simulink model "SpatialContactForceBus"  (R2025a)
settings: Solver=ode45  StartTime=0.0  StopTime=10.0  MaxStep=1e-3  RelTol=1e-3  AbsTol=1e-3
PreLoadFcn:
  | addpath(fullfile('SpatialContactForceBusSupport','Scripts'));
model workspace: external: MATLAB File SpatialContactForceBusParameters.m (data not in the file)
undefined symbols (not defined in the file or in its folder): BackLeft, BackRight, BackStop, Body, car, critical_velocity, damping, EndRamp, FrontLeft, FrontRight, g, Incline, kinetic_friction_coef, LeftRail, Ramp1, Ramp2, Ramp3, Ramp4, ramp_structure, RightRail, static_friction_coef, stiffness, transition_region_width, X, Y, Z
libraries: sm_lib x131, SpatialContactForceBusLibrary x9, nesl_utility x1
(part 1 of 2)
CloseFcn:
  | rmpath(fullfile('SpatialContactForceBusSupport','Scripts'));
Description:
  | Using the Spatial Contact Force Block - Bumper Car
settings Model: Creator=The MathWorks, Inc.  LastModifiedBy=The MathWorks, Inc.
settings SolverCC: AutoScaleAbsTol=off  AlgebraicLoopSolver=TrustRegion
settings DataIOCC: ReturnWorkspaceOutputs=off
settings OptimizationCC: ReuseModelBlockBuffer=off
settings DebuggingCC: UnconnectedInputMsg=warning  UnconnectedOutputMsg=warning  UnconnectedLineMsg=warning  SubsystemReferenceDiagnosticForUnitTest=warning  SymbolicDimsDataTypeCodeGenerationDiagnostic=none
settings ModelReferenceCC: EnableRefExpFcnMdlSchedulingChecks=on
settings RTWCC: GPUComputeCapability=3.5
settings SimscapeCC: SimscapeLogType=all  SimscapeLogSimulationStatistics=on  SimscapeLogName=simlogSpatialContactForceBus  SimscapeLogDataHistory=20000.0
settings ExplorerConfigSet: InternalSimMechanicsExplorerSettings="<ExplorerConfiguration><canonicalview>default</canonicalview><AnimationSetting><BasePlaybackSpeed>1.0</BasePlaybackSpeed><PlaybackSpeedFactor>1.0</PlaybackSpeedFactor></AnimationSetting><TilePanel><TileInfo><Tiles Columns=\"1\" Count=\"1\" Rows=\"1\"><Column Weight=\"1\"/><Row Weight=\"1\"/><Tile Height=\"1\" Width=\"1\" X=\"0\" Y=\"0\"/></Tiles></TileInfo><SceneInfo><SceneViewer><BGColor><R>0.800000011920928955</R><G>0.800000011920928955</G><B>0.800000011920928955</B></BGColor><Camera><DoPerspective>off</DoPerspective><Position><X>0.637508295609907183</X><Y>-0.637508296451667844</Y><Z>1.11601012334107264</Z></Position><Center><X>-0.00639254054797280813</X><Y>0.00639253970621195267</Y><Z>0.472109287183192672</Z></Center><Up><X>-0.408248290463863073</X><Y>0.408248290463863073</Y><Z>0.816496580927726145</Z></Up><ViewLimDist>1</ViewLimDist><YLim>0.759088869094848628</YLim><XLim>0.995304530142192112</XLim></Camera></SceneViewer></SceneInfo></TilePanel><MechEditorPanel><Cameras/><GfxPanelCameraMap/><VideoCreator><PlaybackSpeedRatio>1.0</PlaybackSpeedRatio><FrameRate>30</FrameRate><VideoFormat>Motion JPEG AVI</VideoFormat><FrameSize>auto</FrameSize></VideoCreator></MechEditorPanel></ExplorerConfiguration>"

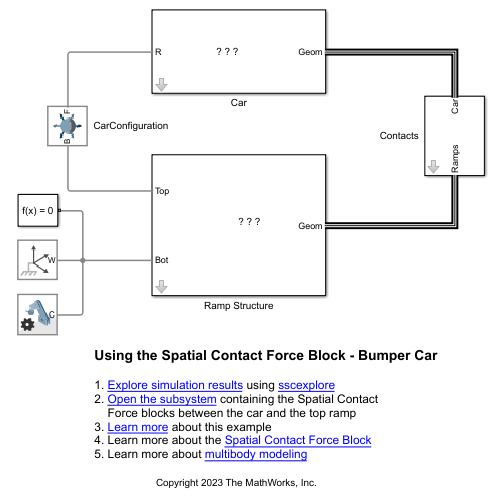
[thumbnail: Simulink's stored preview of the top-level diagram]
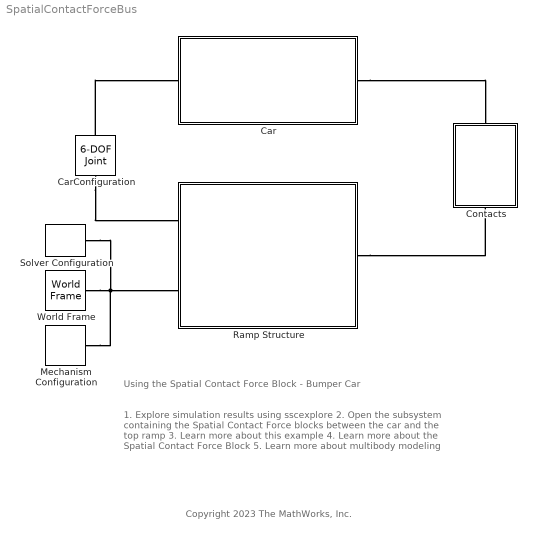
== system SpatialContactForceBus ==
  note: Copyright 2023 The MathWorks, Inc.
  note: Using the Spatial Contact Force Block - Bumper Car
  note: 1. Explore simulation results using sscexplore
      | 2. Open the subsystem containing the Spatial Contact
      | Force blocks between the car and the top ramp
      | 3. Learn more about this example
      | 4. Learn more about the Spatial Contact Force Block
      | 5. Learn more about multibody modeling
  Car : Subsystem  mask{l=car.body.length, w=car.body.width, h=car.body.height, m=car.body.mass, body_color=car.body.color, wheel_radius=car.wheel.radius, wheel_width=car.wheel.thickness, wheel_m=car.wheel.mass, wheel_color=car.wheel.color, wheel_spoke_color=car.wheel.spoke.color}
      mask prompts: l "Length (cm)"; w "Width (cm)"; h "Height (cm)"; m "Body Mass (kg)"; body_color "Car Body Color"; wheel_radius "Radius"; wheel_width "Thickness"; wheel_m "Wheel Mass (kg)"; wheel_color "Wheel Color"; wheel_spoke_color "Wheel Spoke Color"
      mask init:
      | axle_len               = .85 * l;
      | axle_radius            = axle_len / 30;
      | wheel_inner_radius     = .67 * wheel_radius;
      | wheel_spoke_thickness = axle_radius / 2;
      | 
      | front_wheel_pos  = l * .12;
      | back_wheel_pos   = l * .88;
      | wheel_separation = axle_len;
      mask DialogControl BodyGroupVar Prompt: Body
      mask DialogControl BodyDimGroupVar Prompt: Dimensions
      mask DialogControl BodyInertiaGroupVar Prompt: Inertia
      mask DialogControl BodyGraphicGroupVar Prompt: Graphic
      mask DialogControl WheelGroupVar Prompt: Wheels
      mask DialogControl WheelDimGroupVar Prompt: Dimensions
      mask DialogControl WheelInertiaGroupVar Prompt: Inertia
      mask DialogControl WheelGraphicGroupVar Prompt: Graphic
      mask Display: image(fullfile('SpatialContactForceBusSupport','Images','Car.png'));
  CarConfiguration : sm_lib/Joints/6-DOF Joint  JointMode=Normal  CompositeWrenchDir=FollowerOnBase  CompositeWrenchFrame=BaseFrame  SenseConstraintForce=off  SenseConstraintTorque=off  SenseTotalForce=off  SenseTotalTorque=off  PxPositionTargetSpecify=on  PxPositionTargetPriority=High  PxPositionTargetValue=car.start_dist  PxPositionTargetValueUnits=cm  PxVelocityTargetSpecify=off  PxVelocityTargetPriority=High  PxVelocityTargetValue=0  PxVelocityTargetValueUnits=m/s  PxEquilibriumPosition=0  PxEquilibriumPositionUnits=m  PxSpringStiffness=0  PxSpringStiffnessUnits=N/m  PxDampingCoefficient=0  PxDampingCoefficientUnits=N/(m/s)  PxLowerLimitSpecify=off  PxLowerLimitBound=-1  PxLowerLimitBoundUnits=m  PxLowerLimitStiffness=1e6  PxLowerLimitStiffnessUnits=N/m  PxLowerLimitDamping=1e3  PxLowerLimitDampingUnits=N/(m/s)  PxLowerLimitTransitionRegionWidth=1e-4  PxLowerLimitTransitionRegionWidthUnits=m  PxUpperLimitSpecify=off  PxUpperLimitBound=1  PxUpperLimitBoundUnits=m  PxUpperLimitStiffness=1e6  PxUpperLimitStiffnessUnits=N/m  PxUpperLimitDamping=1e3  PxUpperLimitDampingUnits=N/(m/s)  PxUpperLimitTransitionRegionWidth=1e-4  PxUpperLimitTransitionRegionWidthUnits=m  PxTorqueActuationMode=NoTorque  PxMotionActuationMode=ComputedMotion  PxSensePosition=off  PxSenseVelocity=off  PxSenseAcceleration=off  PxSenseTorqueForce=off  PxSenseLowerLimitTorqueForce=off  PxSenseUpperLimitTorqueForce=off  PyPositionTargetSpecify=off  PyPositionTargetPriority=High  PyPositionTargetValue=0  PyPositionTargetValueUnits=m  PyVelocityTargetSpecify=off  PyVelocityTargetPriority=High  PyVelocityTargetValue=0  PyVelocityTargetValueUnits=m/s  PyEquilibriumPosition=0  PyEquilibriumPositionUnits=m  PySpringStiffness=0  PySpringStiffnessUnits=N/m  PyDampingCoefficient=0  PyDampingCoefficientUnits=N/(m/s)  PyLowerLimitSpecify=off  PyLowerLimitBound=-1  PyLowerLimitBoundUnits=m  PyLowerLimitStiffness=1e6  PyLowerLimitStiffnessUnits=N/m  PyLowerLimitDamping=1e3  PyLowerLimitDampingUnits=N/(m/s)  PyLowerLimitTransitionRegionWidth=1e-4  PyLowerLimitTransitionRegionWidthUnits=m  PyUpperLimitSpecify=off  PyUpperLimitBound=1  PyUpperLimitBoundUnits=m  PyUpperLimitStiffness=1e6  PyUpperLimitStiffnessUnits=N/m  PyUpperLimitDamping=1e3  PyUpperLimitDampingUnits=N/(m/s)  PyUpperLimitTransitionRegionWidth=1e-4  PyUpperLimitTransitionRegionWidthUnits=m  PyTorqueActuationMode=NoTorque  PyMotionActuationMode=ComputedMotion  PySensePosition=off  PySenseVelocity=off  PySenseAcceleration=off  PySenseTorqueForce=off  PySenseLowerLimitTorqueForce=off  PySenseUpperLimitTorqueForce=off  PzPositionTargetSpecify=on  PzPositionTargetPriority=High  PzPositionTargetValue=car.start_height  PzPositionTargetValueUnits=cm  PzVelocityTargetSpecify=off  PzVelocityTargetPriority=High  PzVelocityTargetValue=0  PzVelocityTargetValueUnits=m/s  PzEquilibriumPosition=0  PzEquilibriumPositionUnits=m  PzSpringStiffness=0  PzSpringStiffnessUnits=N/m  PzDampingCoefficient=0  PzDampingCoefficientUnits=N/(m/s)  PzLowerLimitSpecify=off  PzLowerLimitBound=-1  PzLowerLimitBoundUnits=m  PzLowerLimitStiffness=1e6  PzLowerLimitStiffnessUnits=N/m  PzLowerLimitDamping=1e3  PzLowerLimitDampingUnits=N/(m/s)  PzLowerLimitTransitionRegionWidth=1e-4  PzLowerLimitTransitionRegionWidthUnits=m  PzUpperLimitSpecify=off  PzUpperLimitBound=1  PzUpperLimitBoundUnits=m  PzUpperLimitStiffness=1e6  PzUpperLimitStiffnessUnits=N/m  PzUpperLimitDamping=1e3  PzUpperLimitDampingUnits=N/(m/s)  PzUpperLimitTransitionRegionWidth=1e-4  PzUpperLimitTransitionRegionWidthUnits=m  PzTorqueActuationMode=NoTorque  PzMotionActuationMode=ComputedMotion  PzSensePosition=off  PzSenseVelocity=off  PzSenseAcceleration=off  PzSenseTorqueForce=off  PzSenseLowerLimitTorqueForce=off  PzSenseUpperLimitTorqueForce=off  SphPositionTargetSpecify=on  SphPositionTargetPriority=High  SphPositionTargetRotationMethod=StandardAxis  SphPositionTargetFollAlignAxisA=+X  SphPositionTargetBaseAlignAxisA=+Y  SphPositionTargetFollAlignAxisB=+Y  SphPositionTargetBaseAlignAxisB=+Z  SphPositionTargetRotationStandardAxis=-Y  SphPositionTargetRotationAngle=car.start_pitch  SphPositionTargetRotationAngleUnits=deg  SphPositionTargetRotationArbitraryAxis=[0 0 1]  SphPositionTargetRotationSequenceAxes=FollowerAxes  SphPositionTargetRotationSequence=XYX  SphPositionTargetRotationSequenceAngles=[0 0 0]  SphPositionTargetRotationSequenceAnglesUnits=deg  SphPositionTargetRotationMatrix=[1 0 0; 0 1 0; 0 0 1]  SphPositionTargetQuaternion=[1 0 0 0]  SphVelocityTargetSpecify=off  SphVelocityTargetPriority=High  SphVelocityTargetValue=[0 0 0]  SphVelocityTargetValueUnits=deg/s  SphVelocityTargetInFollowerFrame=on  SphEqPosRotationMethod=None  SphEqPosFollAlignAxisA=+X  SphEqPosBaseAlignAxisA=+Y  SphEqPosFollAlignAxisB=+Y  SphEqPosBaseAlignAxisB=+Z  SphEqPosRotationStandardAxis=+Z  SphEqPosRotationAngle=0.0  SphEqPosRotationAngleUnits=deg  SphEqPosRotationArbitraryAxis=[0 0 1]  SphEqPosRotationSequenceAxes=FollowerAxes  SphEqPosRotationSequence=XYX  SphEqPosRotationSequenceAngles=[0 0 0]  SphEqPosRotationSequenceAnglesUnits=deg  SphEqPosRotationMatrix=[1 0 0; 0 1 0; 0 0 1]  SphEqPosQuaternion=[1 0 0 0]  SphSpringStiffness=0  SphSpringStiffnessUnits=N*m/deg  SphDampingCoefficient=0  SphDampingCoefficientUnits=N*m/(deg/s)  SphLowerLimitSpecify=off  SphLowerLimitBound=15  SphLowerLimitBoundUnits=deg  SphLowerLimitStiffness=1e4  SphLowerLimitStiffnessUnits=N*m/deg  SphLowerLimitDamping=10  SphLowerLimitDampingUnits=N*m/(deg/s)  SphLowerLimitTransitionRegionWidth=0.1  SphLowerLimitTransitionRegionWidthUnits=deg  SphUpperLimitSpecify=off  SphUpperLimitBound=45  SphUpperLimitBoundUnits=deg  SphUpperLimitStiffness=1e4  SphUpperLimitStiffnessUnits=N*m/deg  SphUpperLimitDamping=10  SphUpperLimitDampingUnits=N*m/(deg/s)  SphUpperLimitTransitionRegionWidth=0.1  SphUpperLimitTransitionRegionWidthUnits=deg  SphTorqueActuationMode=NoTorque  SphActuateTorqueX=off  SphActuateTorqueY=off  SphActuateTorqueZ=off  SphActuateTorque=off  SphActuationFrame=BaseFrame  SphSensePosition=off  SphSenseVelocityX=off  SphSenseVelocityY=off  SphSenseVelocityZ=off  SphSenseVelocity=off  SphSenseAccelerationX=off  SphSenseAccelerationY=off  SphSenseAccelerationZ=off  SphSenseAcceleration=off  SphSenseLowerLimitTorqueMag=off  SphSenseUpperLimitTorqueMag=off  SphSensingFrame=BaseFrame
  Contacts : Subsystem  mask{k=stiffness, b=damping, tau=transition_region_width, mus=static_friction_coef, muk=kinetic_friction_coef, cv=critical_velocity}
      mask prompts: k "Stiffness (N/m)"; b "Damping (N/(m/s))"; tau "Transition Region Width (m)"; mus "Coefficient of Static Friction"; muk "Coefficient of Kinetic Friction"; cv "Critical Velocity (m/s)"
  Mechanism Configuration : sm_lib/Utilities/Mechanism Configuration  UniformGravity=Constant  GravityVector=[0 0 -g]  GravityVectorUnits=m/s^2  LinearizationDelta=0.001  JointModeTransitionNonlinearIterations=2
  Ramp Structure : Subsystem  mask{w=ramp_structure.width, l=ramp_structure.length, ramp_angle=ramp_structure.ramp.angle, surface_color=ramp_structure.ramp.color, rail_color=ramp_structure.rail.color, pillar_color=ramp_structure.pillar.color, base_color=ramp_structure.base.color}
      mask prompts: w "Width (cm)"; l "Length (cm)"; ramp_angle "Ramp Angle (deg)"; surface_color "Surface Color"; rail_color "Rail Color"; pillar_color "Pillar Color"; base_color "Base Color"
      mask init:
      | ramp.angle = ramp_angle;
      | theta_ = deg2rad(ramp.angle);
      | 
      | ramp.w       = w;
      | ramp.h       = ramp.w / 4;
      | 
      | wall.h        = ramp.w;
      | 
      | dropoff_h     = .75 * ramp.w;
      | dropoff_dist  = 1.5 * ramp.w;
      | 
      | ramp.l        = (l - dropoff_dist - sin(theta_)*ramp.h/2)...
      |                 / cos(theta_);
      | 
      | rail.r        = .28 * ramp.h;
      | rail.l        = ramp.l;
      | 
      | rail.h = 1.5 * ramp.h;
      | 
      | end_ramp.l = dropoff_dist + ramp.h;
      | 
      | ramp.w = ramp.w + 2 * rail.r;
      mask DialogControl ParameterGroupVar Prompt: Geometry
      mask DialogControl GraphicsGroupVar Prompt: Graphic
      mask Display: image(fullfile('SpatialContactForceBusSupport','Images','RampStructure.png'));
  Solver Configuration : nesl_utility/Solver Configuration  PhysicalDomain=network_engine_domain  SubClassName=solver  LeftPortType=input  RightPortType=generic  Tones=[]  Harmonics=[]  SimulateNoise=off  Profile=off  UseLocalSampling=off  EnableSwitchedLinearOptims=on  FrequencyDomain=off  UseCCode=off  RelTol=0.001  AbsTol=1e-06  MinStep=1e-09  ToWorkspace=off  RevertToSquareIcSolve=off  NumHomotopyIterations=100  PhasorMode=off  PhasorModeNumHarmonics=1  ConsistencySolver=NEWTON_FTOL  IndexReductionMethod=DerivativeReplacement  DoDC=off  ResidualTolerance=1e-09  ConsistencyTolSource=GLOBAL  ConsistencyAbsTol=0.001  ConsistencyRelTol=0.001  ConsistencyTolFactor=0.001  UseLocalSolver=off  LocalSolverChoice=NE_BACKWARD_EULER_ADVANCER  ResolveIndetEquations=on  FunctionEvalNumThread=1  LocalSolverSampleTime=0.001  DoFixedCost=off  MaxNonlinIter=3  MaxModeIter=2  ComputeImpulses=off  ImpulseIterations=2  LinearAlgebra=Sparse  LinearAlgebraNumThread=0  EquationFormulation=NE_TIME_EF  DelaysMemoryBudget=1024  AutomaticFiltering=on  FilteringTimeConstant=0.001  PartitionStorageMethod=AS_NEEDED  PartitionMemoryBudget=1024  PartitionMethod=FAST  MultibodyUseLocalSolver=off  MultibodyLocalSolverChoice=ODE1  MultibodyLocalSolverSampleTime=0.001
  World Frame : sm_lib/Frames and Transforms/World Frame
  connections:
  Solver Configuration/RConn1 -- Ramp Structure/LConn2 -- Mechanism Configuration/RConn1 -- World Frame/RConn1
  CarConfiguration/RConn1 -- Car/LConn1
  CarConfiguration/LConn1 -- Ramp Structure/LConn1
  Ramp Structure/RConn1 -- Contacts/LConn1
  Car/RConn1 -- Contacts/RConn1

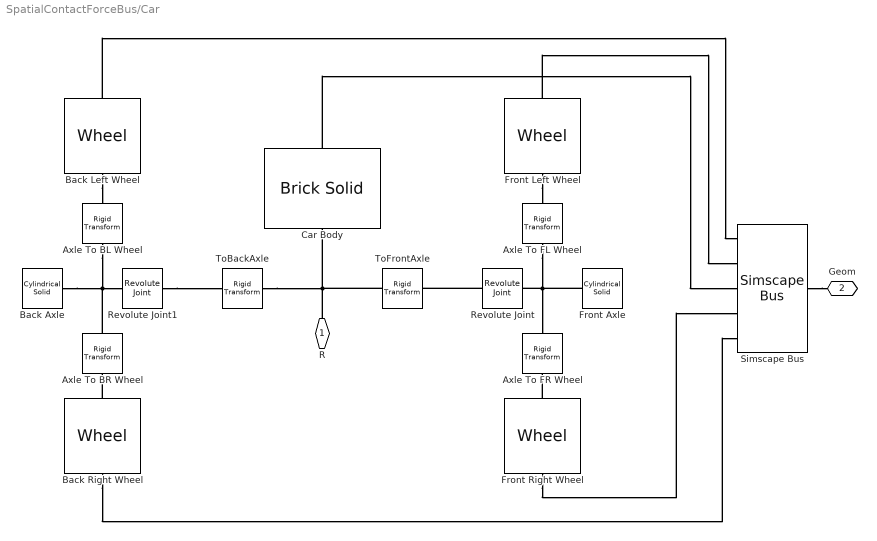
== system SpatialContactForceBus/Car ==
  Axle To BL Wheel : sm_lib/Frames and Transforms/Rigid Transform  RotationMethod=None  FollAlignAxisA=+X  BaseAlignAxisA=+Y  FollAlignAxisB=+Y  BaseAlignAxisB=+Z  RotationStandardAxis=+Z  RotationAngle=0.0  RotationAngleUnits=deg  RotationArbitraryAxis=[0 0 1]  RotationSequenceAxes=FollowerAxes  RotationSequence=XYX  RotationSequenceAngles=[0 0 0]  RotationSequenceAnglesUnits=deg  RotationMatrix=[1 0 0; 0 1 0; 0 0 1]  Quaternion=[1 0 0 0]  TranslationMethod=StandardAxis  TranslationCartesianOffset=[0 0 0]  TranslationCartesianOffsetUnits=cm  TranslationStandardAxis=-Z  TranslationStandardOffset=wheel_separation/2  TranslationStandardOffsetUnits=cm  TranslationROffset=0  TranslationROffsetUnits=m  TranslationThetaOffset=0  TranslationThetaOffsetUnits=deg  TranslationZOffset=0  TranslationZOffsetUnits=m
  Axle To BR Wheel : sm_lib/Frames and Transforms/Rigid Transform  RotationMethod=None  FollAlignAxisA=+X  BaseAlignAxisA=+Y  FollAlignAxisB=+Y  BaseAlignAxisB=+Z  RotationStandardAxis=+Z  RotationAngle=0.0  RotationAngleUnits=deg  RotationArbitraryAxis=[0 0 1]  RotationSequenceAxes=FollowerAxes  RotationSequence=XYX  RotationSequenceAngles=[0 0 0]  RotationSequenceAnglesUnits=deg  RotationMatrix=[1 0 0; 0 1 0; 0 0 1]  Quaternion=[1 0 0 0]  TranslationMethod=StandardAxis  TranslationCartesianOffset=[0 0 0]  TranslationCartesianOffsetUnits=cm  TranslationStandardAxis=+Z  TranslationStandardOffset=wheel_separation/2  TranslationStandardOffsetUnits=cm  TranslationROffset=0  TranslationROffsetUnits=m  TranslationThetaOffset=0  TranslationThetaOffsetUnits=deg  TranslationZOffset=0  TranslationZOffsetUnits=m
  Axle To FL Wheel : sm_lib/Frames and Transforms/Rigid Transform  RotationMethod=None  FollAlignAxisA=+X  BaseAlignAxisA=+Y  FollAlignAxisB=+Y  BaseAlignAxisB=+Z  RotationStandardAxis=+Z  RotationAngle=0.0  RotationAngleUnits=deg  RotationArbitraryAxis=[0 0 1]  RotationSequenceAxes=FollowerAxes  RotationSequence=XYX  RotationSequenceAngles=[0 0 0]  RotationSequenceAnglesUnits=deg  RotationMatrix=[1 0 0; 0 1 0; 0 0 1]  Quaternion=[1 0 0 0]  TranslationMethod=StandardAxis  TranslationCartesianOffset=[0 0 0]  TranslationCartesianOffsetUnits=cm  TranslationStandardAxis=-Z  TranslationStandardOffset=wheel_separation/2  TranslationStandardOffsetUnits=cm  TranslationROffset=0  TranslationROffsetUnits=m  TranslationThetaOffset=0  TranslationThetaOffsetUnits=deg  TranslationZOffset=0  TranslationZOffsetUnits=m
  Axle To FR Wheel : sm_lib/Frames and Transforms/Rigid Transform  RotationMethod=None  FollAlignAxisA=+X  BaseAlignAxisA=+Y  FollAlignAxisB=+Y  BaseAlignAxisB=+Z  RotationStandardAxis=+Z  RotationAngle=0.0  RotationAngleUnits=deg  RotationArbitraryAxis=[0 0 1]  RotationSequenceAxes=FollowerAxes  RotationSequence=XYX  RotationSequenceAngles=[0 0 0]  RotationSequenceAnglesUnits=deg  RotationMatrix=[1 0 0; 0 1 0; 0 0 1]  Quaternion=[1 0 0 0]  TranslationMethod=StandardAxis  TranslationCartesianOffset=[0 0 0]  TranslationCartesianOffsetUnits=cm  TranslationStandardAxis=+Z  TranslationStandardOffset=wheel_separation/2  TranslationStandardOffsetUnits=cm  TranslationROffset=0  TranslationROffsetUnits=m  TranslationThetaOffset=0  TranslationThetaOffsetUnits=deg  TranslationZOffset=0  TranslationZOffsetUnits=m
  Back Axle : sm_lib/Body Elements/Cylindrical Solid  CylinderRadius=axle_radius  CylinderRadiusUnits=cm  CylinderLength=axle_len  CylinderLengthUnits=cm  ExportEntireGeometry=off  InertiaType=CalculateFromGeometry  BasedOnType=Density  Density=0  DensityUnits=kg/m^3  Mass=1  MassUnits=kg  CenterOfMass=[0 0 0]  CenterOfMassUnits=m  MomentsOfInertia=[1 1 1]  MomentsOfInertiaUnits=kg*m^2  ProductsOfInertia=[0 0 0]  ProductsOfInertiaUnits=kg*m^2  GraphicType=FromGeometry  MarkerShape=Sphere  MarkerSize=10  GraphicVisPropType=SimpleVisualProperties  GraphicDiffuseColor=wheel_spoke_color  GraphicOpacity=1.0  GraphicSpecularColor=[0.5 0.5 0.5 1.0]  GraphicAmbientColor=[0.15 0.15 0.15 1.0]  GraphicEmissiveColor=[0.0 0.0 0.0 1.0]  GraphicShininess=75  DoExposeReferenceFrame=on  SerializedFrames=<Frames/>
  Back Left Wheel : SpatialContactForceBusLibrary/Wheel  r=wheel_radius  rin=wheel_inner_radius  spoke_r=wheel_spoke_thickness  W=wheel_width  m=wheel_m  color=wheel_color  spoke_color=wheel_spoke_color
  Back Right Wheel : SpatialContactForceBusLibrary/Wheel  r=wheel_radius  rin=wheel_inner_radius  spoke_r=wheel_spoke_thickness  W=wheel_width  m=wheel_m  color=wheel_color  spoke_color=wheel_spoke_color
  Car Body : sm_lib/Body Elements/Brick Solid  BrickDimensions=[l w h]  BrickDimensionsUnits=cm  ExportEntireGeometry=on  InertiaType=CalculateFromGeometry  BasedOnType=Mass  Density=1000  DensityUnits=kg/m^3  Mass=m  MassUnits=kg  CenterOfMass=[0 0 0]  CenterOfMassUnits=cm  MomentsOfInertia=[1 1 1]  MomentsOfInertiaUnits=kg*m^2  ProductsOfInertia=[0 0 0]  ProductsOfInertiaUnits=kg*m^2  GraphicType=FromGeometry  MarkerShape=Sphere  MarkerSize=10  GraphicVisPropType=SimpleVisualProperties  GraphicDiffuseColor=body_color  GraphicOpacity=1.0  GraphicSpecularColor=[0.5 0.5 0.5 1.0]  GraphicAmbientColor=[0.15 0.15 0.15 1.0]  GraphicEmissiveColor=[0.0 0.0 0.0 1.0]  GraphicShininess=75  DoExposeReferenceFrame=on  SerializedFrames=<Frames/>
  Front Axle : sm_lib/Body Elements/Cylindrical Solid  CylinderRadius=axle_radius  CylinderRadiusUnits=cm  CylinderLength=axle_len  CylinderLengthUnits=cm  ExportEntireGeometry=off  InertiaType=CalculateFromGeometry  BasedOnType=Density  Density=0  DensityUnits=kg/m^3  Mass=1  MassUnits=kg  CenterOfMass=[0 0 0]  CenterOfMassUnits=m  MomentsOfInertia=[1 1 1]  MomentsOfInertiaUnits=kg*m^2  ProductsOfInertia=[0 0 0]  ProductsOfInertiaUnits=kg*m^2  GraphicType=FromGeometry  MarkerShape=Sphere  MarkerSize=10  GraphicVisPropType=SimpleVisualProperties  GraphicDiffuseColor=wheel_spoke_color  GraphicOpacity=1.0  GraphicSpecularColor=[0.5 0.5 0.5 1.0]  GraphicAmbientColor=[0.15 0.15 0.15 1.0]  GraphicEmissiveColor=[0.0 0.0 0.0 1.0]  GraphicShininess=75  DoExposeReferenceFrame=on  SerializedFrames=<Frames/>
  Front Left Wheel : SpatialContactForceBusLibrary/Wheel  r=wheel_radius  rin=wheel_inner_radius  spoke_r=wheel_spoke_thickness  W=wheel_width  m=wheel_m  color=wheel_color  spoke_color=wheel_spoke_color
  Front Right Wheel : SpatialContactForceBusLibrary/Wheel  r=wheel_radius  rin=wheel_inner_radius  spoke_r=wheel_spoke_thickness  W=wheel_width  m=wheel_m  color=wheel_color  spoke_color=wheel_spoke_color
  Revolute Joint : sm_lib/Joints/Revolute Joint  JointMode=Normal  CompositeWrenchDir=FollowerOnBase  CompositeWrenchFrame=BaseFrame  SenseConstraintForce=off  SenseConstraintTorque=off  SenseTotalForce=off  SenseTotalTorque=off  PositionTargetSpecify=off  PositionTargetPriority=High  PositionTargetValue=0  PositionTargetValueUnits=deg  VelocityTargetSpecify=off  VelocityTargetPriority=High  VelocityTargetValue=0  VelocityTargetValueUnits=deg/s  EquilibriumPosition=0  EquilibriumPositionUnits=deg  SpringStiffness=0  SpringStiffnessUnits=N*m/deg  DampingCoefficient=0  DampingCoefficientUnits=N*m/(deg/s)  LowerLimitSpecify=off  LowerLimitBound=-90  LowerLimitBoundUnits=deg  LowerLimitStiffness=1e4  LowerLimitStiffnessUnits=N*m/deg  LowerLimitDamping=10  LowerLimitDampingUnits=N*m/(deg/s)  LowerLimitTransitionRegionWidth=0.1  LowerLimitTransitionRegionWidthUnits=deg  UpperLimitSpecify=off  UpperLimitBound=90  UpperLimitBoundUnits=deg  UpperLimitStiffness=1e4  UpperLimitStiffnessUnits=N*m/deg  UpperLimitDamping=10  UpperLimitDampingUnits=N*m/(deg/s)  UpperLimitTransitionRegionWidth=0.1  UpperLimitTransitionRegionWidthUnits=deg  TorqueActuationMode=NoTorque  MotionActuationMode=ComputedMotion  SensePosition=off  SenseVelocity=off  SenseAcceleration=off  SenseTorqueForce=off  SenseLowerLimitTorqueForce=off  SenseUpperLimitTorqueForce=off
  Revolute Joint1 : sm_lib/Joints/Revolute Joint  JointMode=Normal  CompositeWrenchDir=FollowerOnBase  CompositeWrenchFrame=BaseFrame  SenseConstraintForce=off  SenseConstraintTorque=off  SenseTotalForce=off  SenseTotalTorque=off  PositionTargetSpecify=off  PositionTargetPriority=High  PositionTargetValue=0  PositionTargetValueUnits=deg  VelocityTargetSpecify=off  VelocityTargetPriority=High  VelocityTargetValue=0  VelocityTargetValueUnits=deg/s  EquilibriumPosition=0  EquilibriumPositionUnits=deg  SpringStiffness=0  SpringStiffnessUnits=N*m/deg  DampingCoefficient=0  DampingCoefficientUnits=N*m/(deg/s)  LowerLimitSpecify=off  LowerLimitBound=-90  LowerLimitBoundUnits=deg  LowerLimitStiffness=1e4  LowerLimitStiffnessUnits=N*m/deg  LowerLimitDamping=10  LowerLimitDampingUnits=N*m/(deg/s)  LowerLimitTransitionRegionWidth=0.1  LowerLimitTransitionRegionWidthUnits=deg  UpperLimitSpecify=off  UpperLimitBound=90  UpperLimitBoundUnits=deg  UpperLimitStiffness=1e4  UpperLimitStiffnessUnits=N*m/deg  UpperLimitDamping=10  UpperLimitDampingUnits=N*m/(deg/s)  UpperLimitTransitionRegionWidth=0.1  UpperLimitTransitionRegionWidthUnits=deg  TorqueActuationMode=NoTorque  MotionActuationMode=ComputedMotion  SensePosition=off  SenseVelocity=off  SenseAcceleration=off  SenseTorqueForce=off  SenseLowerLimitTorqueForce=off  SenseUpperLimitTorqueForce=off
  Simscape Bus : SimscapeBus  HierarchyStrings=BackLeft;FrontLeft;Body;FrontRight;BackRight
  ToBackAxle : sm_lib/Frames and Transforms/Rigid Transform  RotationMethod=AlignedAxes  FollAlignAxisA=+Y  BaseAlignAxisA=+Z  FollAlignAxisB=+Z  BaseAlignAxisB=-Y  RotationStandardAxis=+Z  RotationAngle=0.0  RotationAngleUnits=deg  RotationArbitraryAxis=[0 0 1]  RotationSequenceAxes=FollowerAxes  RotationSequence=XYX  RotationSequenceAngles=[0 0 0]  RotationSequenceAnglesUnits=deg  RotationMatrix=[1 0 0; 0 1 0; 0 0 1]  Quaternion=[1 0 0 0]  TranslationMethod=StandardAxis  TranslationCartesianOffset=[0 0 0]  TranslationCartesianOffsetUnits=cm  TranslationStandardAxis=+X  TranslationStandardOffset=l/2 - back_wheel_pos  TranslationStandardOffsetUnits=cm  TranslationROffset=0  TranslationROffsetUnits=m  TranslationThetaOffset=0  TranslationThetaOffsetUnits=deg  TranslationZOffset=0  TranslationZOffsetUnits=m
  ToFrontAxle : sm_lib/Frames and Transforms/Rigid Transform  RotationMethod=AlignedAxes  FollAlignAxisA=+Y  BaseAlignAxisA=+Z  FollAlignAxisB=+Z  BaseAlignAxisB=-Y  RotationStandardAxis=+Z  RotationAngle=0.0  RotationAngleUnits=deg  RotationArbitraryAxis=[0 0 1]  RotationSequenceAxes=FollowerAxes  RotationSequence=XYX  RotationSequenceAngles=[0 0 0]  RotationSequenceAnglesUnits=deg  RotationMatrix=[1 0 0; 0 1 0; 0 0 1]  Quaternion=[1 0 0 0]  TranslationMethod=StandardAxis  TranslationCartesianOffset=[0 0 0]  TranslationCartesianOffsetUnits=cm  TranslationStandardAxis=+X  TranslationStandardOffset=l/2 - front_wheel_pos  TranslationStandardOffsetUnits=cm  TranslationROffset=0  TranslationROffsetUnits=m  TranslationThetaOffset=0  TranslationThetaOffsetUnits=deg  TranslationZOffset=0  TranslationZOffsetUnits=m
  R : PMIOPort  Side=Left
  Geom : PMIOPort  Port=2  Side=Right
  connections:
  Back Right Wheel/LConn1 -- Axle To BR Wheel/RConn1
  ToFrontAxle/LConn1 -- Car Body/RConn1 -- R/RConn1 -- ToBackAxle/LConn1
  Front Left Wheel/LConn1 -- Axle To FL Wheel/RConn1
  Revolute Joint1/LConn1 -- ToBackAxle/RConn1
  Revolute Joint/LConn1 -- ToFrontAxle/RConn1
  Axle To FL Wheel/LConn1 -- Front Axle/RConn1 -- Axle To FR Wheel/LConn1 -- Revolute Joint/RConn1
  Axle To BR Wheel/LConn1 -- Back Axle/RConn1 -- Axle To BL Wheel/LConn1 -- Revolute Joint1/RConn1
  Front Right Wheel/LConn1 -- Axle To FR Wheel/RConn1
  Back Left Wheel/LConn1 -- Axle To BL Wheel/RConn1
  Simscape Bus/RConn1 -- Geom/RConn1
  Car Body/LConn1 -- Simscape Bus/LConn3
  Front Left Wheel/RConn1 -- Simscape Bus/LConn2
  Back Left Wheel/RConn1 -- Simscape Bus/LConn1
  Front Right Wheel/RConn1 -- Simscape Bus/LConn4
  Back Right Wheel/RConn1 -- Simscape Bus/LConn5

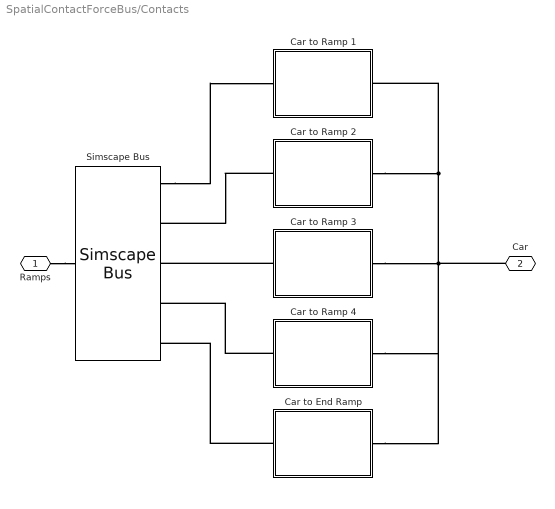
== system SpatialContactForceBus/Contacts ==
  Car to End Ramp : Subsystem
  Car to Ramp 1 : Subsystem
  Car to Ramp 2 : Subsystem
  Car to Ramp 3 : Subsystem
  Car to Ramp 4 : Subsystem
  Simscape Bus : SimscapeBus  HierarchyStrings=Ramp1;Ramp2;Ramp3;Ramp4;EndRamp
  Ramps : PMIOPort  Side=Left
  Car : PMIOPort  Port=2  Side=Right
  connections:
  Ramps/RConn1 -- Simscape Bus/RConn1
  Simscape Bus/LConn1 -- Car to Ramp 1/LConn1
  Car to Ramp 2/LConn1 -- Simscape Bus/LConn2
  Car to Ramp 3/LConn1 -- Simscape Bus/LConn3
  Car to Ramp 4/LConn1 -- Simscape Bus/LConn4
  Car to End Ramp/LConn1 -- Simscape Bus/LConn5
  Car/RConn1 -- Car to Ramp 3/RConn1 -- Car to End Ramp/RConn1 -- Car to Ramp 4/RConn1 -- Car to Ramp 2/RConn1 -- Car to Ramp 1/RConn1

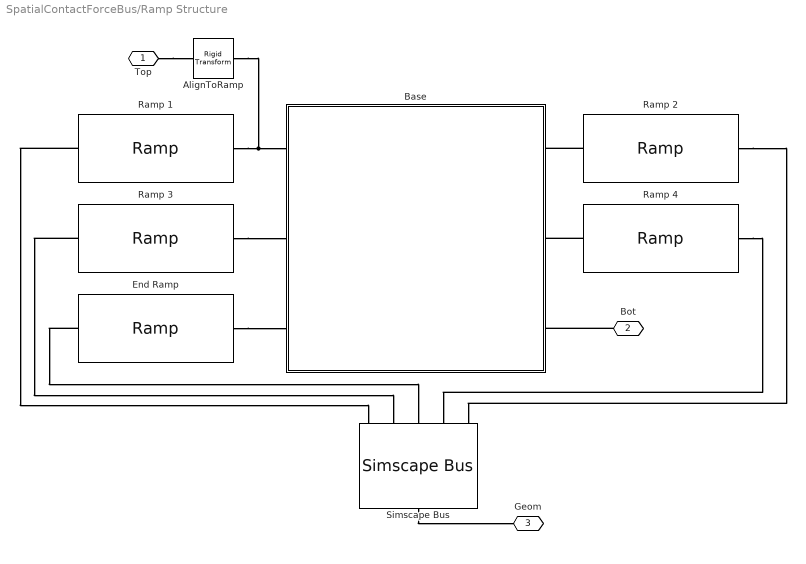
== system SpatialContactForceBus/Ramp Structure ==
  AlignToRamp : sm_lib/Frames and Transforms/Rigid Transform  RotationMethod=StandardAxis  FollAlignAxisA=+X  BaseAlignAxisA=+Y  FollAlignAxisB=+Y  BaseAlignAxisB=+Z  RotationStandardAxis=+Y  RotationAngle=ramp_angle  RotationAngleUnits=deg  RotationArbitraryAxis=[0 0 1]  RotationSequenceAxes=FollowerAxes  RotationSequence=XYX  RotationSequenceAngles=[0 0 0]  RotationSequenceAnglesUnits=deg  RotationMatrix=[1 0 0; 0 1 0; 0 0 1]  Quaternion=[1 0 0 0]  TranslationMethod=None  TranslationCartesianOffset=[0 0 0]  TranslationCartesianOffsetUnits=cm  TranslationStandardAxis=+Z  TranslationStandardOffset=0  TranslationStandardOffsetUnits=cm  TranslationROffset=0  TranslationROffsetUnits=m  TranslationThetaOffset=0  TranslationThetaOffsetUnits=deg  TranslationZOffset=0  TranslationZOffsetUnits=m
  Base : Subsystem  mask{width=w, length=l, ramp_length=ramp.l, ramp_width=ramp.w, ramp_height=ramp.h, backstop_height=wall.h, ramp_angle=ramp.angle, rail_radius=rail.r, dropoff_height=dropoff_h}
      mask prompts: width "Width (cm)"; length "Length (cm)"; ramp_length "Ramp Length (cm)"; ramp_width "Ramp Width (cm)"; ramp_height "Ramp Height (cm)"; backstop_height "Back Stop Height (cm)"; ramp_angle "Ramp Angle (degrees)"; rail_radius "Rail Radius (cm)"; dropoff_height "Dropoff Height (cm)"
      mask init:
      | theta_ = deg2rad(ramp_angle);
      | 
      | ramp_vert_height    = ramp_length * sin(theta_);
      | 
      | pillar_height       = 4 * ramp_vert_height...
      |                       + 3 * dropoff_height...
      |                       + 4 * ramp_height;
      | 
      | pillar_width        = 2.2 * rail_radius;
      | contraption_length  = length;      % distance between opposite support
      |                                    % pillars
      | base_length         = contraption_length + 15;
      | base_width          = ramp_width + 4 * pillar_width;
      | base_height         = .28 * width;
      mask Display: image(fullfile('SpatialContactForceBusSupport','Images','Pillars.png'));
  End Ramp : SpatialContactForceBusLibrary/Ramp  L=end_ramp.l  W=ramp.w  H=ramp.h  wall_h=wall.h  incline=0  rail_r=rail.r  rail_l=end_ramp.l  rail_h=rail.h  color=surface_color  rail_color=rail_color
  Ramp {1..4} (4 alike) : SpatialContactForceBusLibrary/Ramp  L=ramp.l  W=ramp.w  H=ramp.h  wall_h=wall.h  incline=ramp.angle  rail_r=rail.r  rail_l=rail.l  rail_h=rail.h  color=surface_color  rail_color=rail_color
  Simscape Bus : SimscapeBus  HierarchyStrings=Ramp1;Ramp3;EndRamp;Ramp4;Ramp2
  Top : PMIOPort  Side=Left
  Bot : PMIOPort  Port=2  Side=Left
  Geom : PMIOPort  Port=3  Side=Right
  connections:
  Simscape Bus/RConn1 -- Geom/RConn1
  Top/RConn1 -- AlignToRamp/RConn1
  Bot/RConn1 -- Base/RConn3
  Ramp 4/LConn1 -- Base/RConn2
  Ramp 2/LConn1 -- Base/RConn1
  End Ramp/LConn1 -- Base/LConn3
  Ramp 3/LConn1 -- Base/LConn2
  Ramp 1/LConn1 -- AlignToRamp/LConn1 -- Base/LConn1
  Ramp 4/RConn1 -- Simscape Bus/LConn4
  Ramp 1/RConn1 -- Simscape Bus/LConn1
  Ramp 3/RConn1 -- Simscape Bus/LConn2
  End Ramp/RConn1 -- Simscape Bus/LConn3
  Ramp 2/RConn1 -- Simscape Bus/LConn5

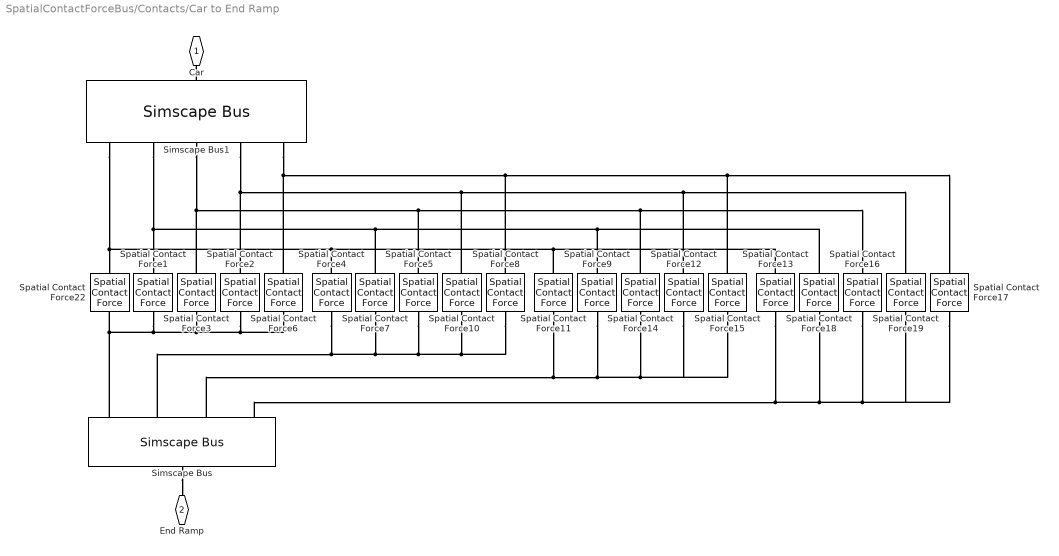
== system SpatialContactForceBus/Contacts/Car to End Ramp ==
  Simscape Bus : SimscapeBus  HierarchyStrings=Incline;BackStop;LeftRail;RightRail
  Simscape Bus1 : SimscapeBus  HierarchyStrings=Body;BackLeft;BackRight;FrontLeft;FrontRight
  Spatial Contact Force{1..19,22} (20 alike) : sm_lib/Forces and Torques/Spatial Contact Force  SenseSeparationDistance=off  NormalForceType=SmoothSpringDamper  NormalStiffness=k  NormalStiffnessUnits=N/m  NormalDamping=b  NormalDampingUnits=N/(m/s)  NormalTransitionRegionWidth=tau  NormalTransitionRegionWidthUnits=m  FrictionType=SmoothStickSlip  CoefficientOfStaticFriction=mus  CoefficientOfDynamicFriction=muk  FrictionalCriticalVelocity=cv  FrictionalCriticalVelocityUnits=m/s  SenseContactSignal=off  SensePenetrationDepth=off  SenseNormalVelocity=off  SenseTangentialVelocity=off  SensingForceTorqueDirection=BaseOnFollower  SensingForceTorqueResolutionFrame=ContactFrame  SenseNormalForce=off  SenseNormalForceMagnitude=off  SenseNormalTorque=off  SenseFrictionalForce=off  SenseFrictionalForceMagnitude=off  SenseFrictionalTorque=off  SenseTotalForce=off  SenseTotalTorque=off  SenseContactBaseRotation=off  SenseContactBaseTranslation=off  SenseContactFollowerRotation=off  SenseContactFollowerTranslation=off  ZeroCrossDetectContactStartAndEnd=off
  Car : PMIOPort  Side=Right
  End Ramp : PMIOPort  Port=2  Side=Left
  connections:
  Simscape Bus1/LConn5 -- Spatial Contact Force6/RConn1 -- Spatial Contact Force8/RConn1 -- Spatial Contact Force17/RConn1 -- Spatial Contact Force15/RConn1
  Spatial Contact Force2/RConn1 -- Simscape Bus1/LConn4 -- Spatial Contact Force10/RConn1 -- Spatial Contact Force19/RConn1 -- Spatial Contact Force12/RConn1
  Spatial Contact Force3/RConn1 -- Spatial Contact Force5/RConn1 -- Spatial Contact Force14/RConn1 -- Spatial Contact Force16/RConn1 -- Simscape Bus1/LConn3
  Spatial Contact Force18/RConn1 -- Spatial Contact Force9/RConn1 -- Spatial Contact Force7/RConn1 -- Simscape Bus1/LConn2 -- Spatial Contact Force1/RConn1
  Spatial Contact Force11/RConn1 -- Spatial Contact Force13/RConn1 -- Spatial Contact Force4/RConn1 -- Simscape Bus1/LConn1 -- Spatial Contact Force22/RConn1
  Simscape Bus1/RConn1 -- Car/RConn1
  Simscape Bus/RConn1 -- End Ramp/RConn1
  Spatial Contact Force18/LConn1 -- Spatial Contact Force17/LConn1 -- Spatial Contact Force19/LConn1 -- Spatial Contact Force16/LConn1 -- Spatial Contact Force13/LConn1 -- Simscape Bus/LConn4
  Spatial Contact Force11/LConn1 -- Simscape Bus/LConn3 -- Spatial Contact Force9/LConn1 -- Spatial Contact Force15/LConn1 -- Spatial Contact Force12/LConn1 -- Spatial Contact Force14/LConn1
  Spatial Contact Force10/LConn1 -- Spatial Contact Force8/LConn1 -- Spatial Contact Force5/LConn1 -- Spatial Contact Force7/LConn1 -- Spatial Contact Force4/LConn1 -- Simscape Bus/LConn2
  Spatial Contact Force2/LConn1 -- Spatial Contact Force6/LConn1 -- Simscape Bus/LConn1 -- Spatial Contact Force22/LConn1 -- Spatial Contact Force1/LConn1 -- Spatial Contact Force3/LConn1

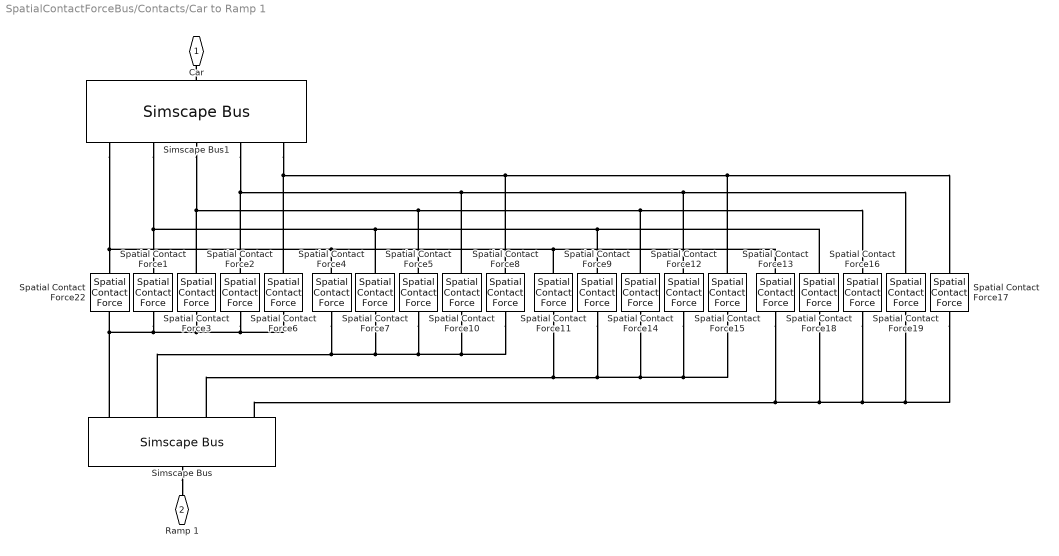
== system SpatialContactForceBus/Contacts/Car to Ramp 1 ==
  Simscape Bus : SimscapeBus  HierarchyStrings=Incline;BackStop;LeftRail;RightRail
  Simscape Bus1 : SimscapeBus  HierarchyStrings=Body;BackLeft;BackRight;FrontLeft;FrontRight
  Spatial Contact Force{1..19,22} (20 alike) : sm_lib/Forces and Torques/Spatial Contact Force  SenseSeparationDistance=off  NormalForceType=SmoothSpringDamper  NormalStiffness=k  NormalStiffnessUnits=N/m  NormalDamping=b  NormalDampingUnits=N/(m/s)  NormalTransitionRegionWidth=tau  NormalTransitionRegionWidthUnits=m  FrictionType=SmoothStickSlip  CoefficientOfStaticFriction=mus  CoefficientOfDynamicFriction=muk  FrictionalCriticalVelocity=cv  FrictionalCriticalVelocityUnits=m/s  SenseContactSignal=off  SensePenetrationDepth=off  SenseNormalVelocity=off  SenseTangentialVelocity=off  SensingForceTorqueDirection=BaseOnFollower  SensingForceTorqueResolutionFrame=ContactFrame  SenseNormalForce=off  SenseNormalForceMagnitude=off  SenseNormalTorque=off  SenseFrictionalForce=off  SenseFrictionalForceMagnitude=off  SenseFrictionalTorque=off  SenseTotalForce=off  SenseTotalTorque=off  SenseContactBaseRotation=off  SenseContactBaseTranslation=off  SenseContactFollowerRotation=off  SenseContactFollowerTranslation=off  ZeroCrossDetectContactStartAndEnd=off
  Car : PMIOPort  Side=Right
  Ramp 1 : PMIOPort  Port=2  Side=Left
  connections:
  Spatial Contact Force22/LConn1 -- Simscape Bus/LConn1 -- Spatial Contact Force6/LConn1 -- Spatial Contact Force2/LConn1 -- Spatial Contact Force3/LConn1 -- Spatial Contact Force1/LConn1
  Simscape Bus/LConn2 -- Spatial Contact Force10/LConn1 -- Spatial Contact Force8/LConn1 -- Spatial Contact Force5/LConn1 -- Spatial Contact Force7/LConn1 -- Spatial Contact Force4/LConn1
  Simscape Bus/LConn3 -- Spatial Contact Force11/LConn1 -- Spatial Contact Force14/LConn1 -- Spatial Contact Force12/LConn1 -- Spatial Contact Force15/LConn1 -- Spatial Contact Force9/LConn1
  Simscape Bus/LConn4 -- Spatial Contact Force18/LConn1 -- Spatial Contact Force16/LConn1 -- Spatial Contact Force19/LConn1 -- Spatial Contact Force17/LConn1 -- Spatial Contact Force13/LConn1
  Simscape Bus/RConn1 -- Ramp 1/RConn1
  Simscape Bus1/RConn1 -- Car/RConn1
  Simscape Bus1/LConn1 -- Spatial Contact Force13/RConn1 -- Spatial Contact Force11/RConn1 -- Spatial Contact Force4/RConn1 -- Spatial Contact Force22/RConn1
  Simscape Bus1/LConn2 -- Spatial Contact Force9/RConn1 -- Spatial Contact Force18/RConn1 -- Spatial Contact Force7/RConn1 -- Spatial Contact Force1/RConn1
  Simscape Bus1/LConn3 -- Spatial Contact Force3/RConn1 -- Spatial Contact Force16/RConn1 -- Spatial Contact Force14/RConn1 -- Spatial Contact Force5/RConn1
  Simscape Bus1/LConn4 -- Spatial Contact Force2/RConn1 -- Spatial Contact Force12/RConn1 -- Spatial Contact Force19/RConn1 -- Spatial Contact Force10/RConn1
  Simscape Bus1/LConn5 -- Spatial Contact Force15/RConn1 -- Spatial Contact Force17/RConn1 -- Spatial Contact Force8/RConn1 -- Spatial Contact Force6/RConn1

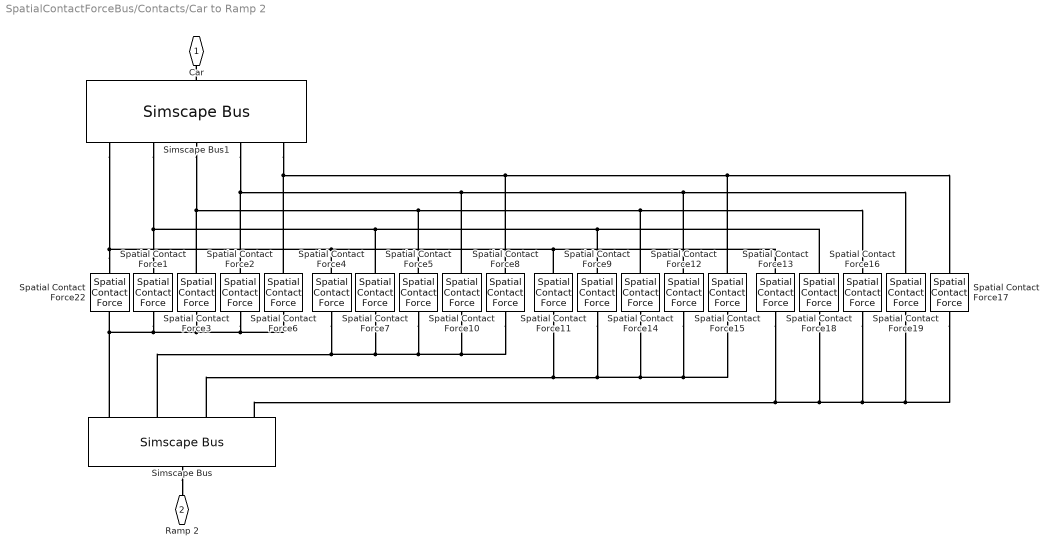
== system SpatialContactForceBus/Contacts/Car to Ramp 2 ==
  Simscape Bus : SimscapeBus  HierarchyStrings=Incline;BackStop;LeftRail;RightRail
  Simscape Bus1 : SimscapeBus  HierarchyStrings=Body;BackLeft;BackRight;FrontLeft;FrontRight
  Spatial Contact Force{1..19,22} (20 alike) : sm_lib/Forces and Torques/Spatial Contact Force  SenseSeparationDistance=off  NormalForceType=SmoothSpringDamper  NormalStiffness=k  NormalStiffnessUnits=N/m  NormalDamping=b  NormalDampingUnits=N/(m/s)  NormalTransitionRegionWidth=tau  NormalTransitionRegionWidthUnits=m  FrictionType=SmoothStickSlip  CoefficientOfStaticFriction=mus  CoefficientOfDynamicFriction=muk  FrictionalCriticalVelocity=cv  FrictionalCriticalVelocityUnits=m/s  SenseContactSignal=off  SensePenetrationDepth=off  SenseNormalVelocity=off  SenseTangentialVelocity=off  SensingForceTorqueDirection=BaseOnFollower  SensingForceTorqueResolutionFrame=ContactFrame  SenseNormalForce=off  SenseNormalForceMagnitude=off  SenseNormalTorque=off  SenseFrictionalForce=off  SenseFrictionalForceMagnitude=off  SenseFrictionalTorque=off  SenseTotalForce=off  SenseTotalTorque=off  SenseContactBaseRotation=off  SenseContactBaseTranslation=off  SenseContactFollowerRotation=off  SenseContactFollowerTranslation=off  ZeroCrossDetectContactStartAndEnd=off
  Car : PMIOPort  Side=Right
  Ramp 2 : PMIOPort  Port=2  Side=Left
  connections:
  Spatial Contact Force3/LConn1 -- Spatial Contact Force1/LConn1 -- Spatial Contact Force22/LConn1 -- Simscape Bus/LConn1 -- Spatial Contact Force6/LConn1 -- Spatial Contact Force2/LConn1
  Simscape Bus/LConn2 -- Spatial Contact Force4/LConn1 -- Spatial Contact Force7/LConn1 -- Spatial Contact Force5/LConn1 -- Spatial Contact Force8/LConn1 -- Spatial Contact Force10/LConn1
  Spatial Contact Force14/LConn1 -- Spatial Contact Force12/LConn1 -- Spatial Contact Force15/LConn1 -- Spatial Contact Force9/LConn1 -- Simscape Bus/LConn3 -- Spatial Contact Force11/LConn1
  Simscape Bus/LConn4 -- Spatial Contact Force13/LConn1 -- Spatial Contact Force16/LConn1 -- Spatial Contact Force19/LConn1 -- Spatial Contact Force17/LConn1 -- Spatial Contact Force18/LConn1
  Simscape Bus/RConn1 -- Ramp 2/RConn1
  Simscape Bus1/RConn1 -- Car/RConn1
  Spatial Contact Force22/RConn1 -- Simscape Bus1/LConn1 -- Spatial Contact Force4/RConn1 -- Spatial Contact Force13/RConn1 -- Spatial Contact Force11/RConn1
  Spatial Contact Force1/RConn1 -- Simscape Bus1/LConn2 -- Spatial Contact Force7/RConn1 -- Spatial Contact Force9/RConn1 -- Spatial Contact Force18/RConn1
  Simscape Bus1/LConn3 -- Spatial Contact Force16/RConn1 -- Spatial Contact Force14/RConn1 -- Spatial Contact Force5/RConn1 -- Spatial Contact Force3/RConn1
  Spatial Contact Force12/RConn1 -- Spatial Contact Force19/RConn1 -- Spatial Contact Force10/RConn1 -- Simscape Bus1/LConn4 -- Spatial Contact Force2/RConn1
  Spatial Contact Force15/RConn1 -- Spatial Contact Force17/RConn1 -- Spatial Contact Force8/RConn1 -- Spatial Contact Force6/RConn1 -- Simscape Bus1/LConn5

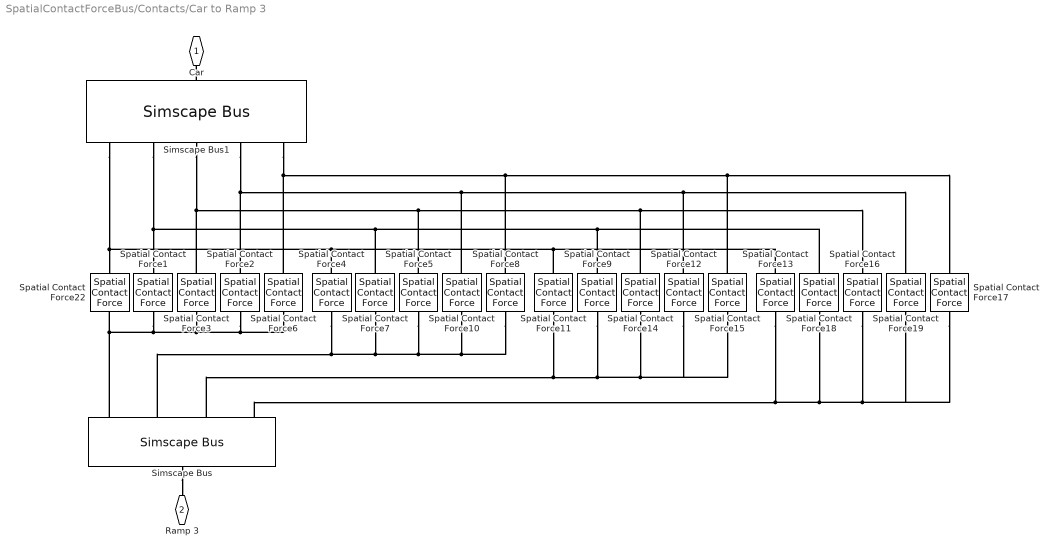
== system SpatialContactForceBus/Contacts/Car to Ramp 3 ==
  Simscape Bus : SimscapeBus  HierarchyStrings=Incline;BackStop;LeftRail;RightRail
  Simscape Bus1 : SimscapeBus  HierarchyStrings=Body;BackLeft;BackRight;FrontLeft;FrontRight
  Spatial Contact Force{1..19,22} (20 alike) : sm_lib/Forces and Torques/Spatial Contact Force  SenseSeparationDistance=off  NormalForceType=SmoothSpringDamper  NormalStiffness=k  NormalStiffnessUnits=N/m  NormalDamping=b  NormalDampingUnits=N/(m/s)  NormalTransitionRegionWidth=tau  NormalTransitionRegionWidthUnits=m  FrictionType=SmoothStickSlip  CoefficientOfStaticFriction=mus  CoefficientOfDynamicFriction=muk  FrictionalCriticalVelocity=cv  FrictionalCriticalVelocityUnits=m/s  SenseContactSignal=off  SensePenetrationDepth=off  SenseNormalVelocity=off  SenseTangentialVelocity=off  SensingForceTorqueDirection=BaseOnFollower  SensingForceTorqueResolutionFrame=ContactFrame  SenseNormalForce=off  SenseNormalForceMagnitude=off  SenseNormalTorque=off  SenseFrictionalForce=off  SenseFrictionalForceMagnitude=off  SenseFrictionalTorque=off  SenseTotalForce=off  SenseTotalTorque=off  SenseContactBaseRotation=off  SenseContactBaseTranslation=off  SenseContactFollowerRotation=off  SenseContactFollowerTranslation=off  ZeroCrossDetectContactStartAndEnd=off
  Car : PMIOPort  Side=Right
  Ramp 3 : PMIOPort  Port=2  Side=Left
  connections:
  Simscape Bus1/LConn5 -- Spatial Contact Force6/RConn1 -- Spatial Contact Force8/RConn1 -- Spatial Contact Force17/RConn1 -- Spatial Contact Force15/RConn1
  Spatial Contact Force2/RConn1 -- Simscape Bus1/LConn4 -- Spatial Contact Force10/RConn1 -- Spatial Contact Force19/RConn1 -- Spatial Contact Force12/RConn1
  Spatial Contact Force3/RConn1 -- Spatial Contact Force5/RConn1 -- Spatial Contact Force14/RConn1 -- Spatial Contact Force16/RConn1 -- Simscape Bus1/LConn3
  Spatial Contact Force18/RConn1 -- Spatial Contact Force9/RConn1 -- Spatial Contact Force7/RConn1 -- Simscape Bus1/LConn2 -- Spatial Contact Force1/RConn1
  Spatial Contact Force11/RConn1 -- Spatial Contact Force13/RConn1 -- Spatial Contact Force4/RConn1 -- Simscape Bus1/LConn1 -- Spatial Contact Force22/RConn1
  Simscape Bus1/RConn1 -- Car/RConn1
  Simscape Bus/RConn1 -- Ramp 3/RConn1
  Spatial Contact Force18/LConn1 -- Spatial Contact Force17/LConn1 -- Spatial Contact Force19/LConn1 -- Spatial Contact Force16/LConn1 -- Spatial Contact Force13/LConn1 -- Simscape Bus/LConn4
  Spatial Contact Force11/LConn1 -- Simscape Bus/LConn3 -- Spatial Contact Force9/LConn1 -- Spatial Contact Force15/LConn1 -- Spatial Contact Force12/LConn1 -- Spatial Contact Force14/LConn1
  Spatial Contact Force10/LConn1 -- Spatial Contact Force8/LConn1 -- Spatial Contact Force5/LConn1 -- Spatial Contact Force7/LConn1 -- Spatial Contact Force4/LConn1 -- Simscape Bus/LConn2
  Spatial Contact Force2/LConn1 -- Spatial Contact Force6/LConn1 -- Simscape Bus/LConn1 -- Spatial Contact Force22/LConn1 -- Spatial Contact Force1/LConn1 -- Spatial Contact Force3/LConn1

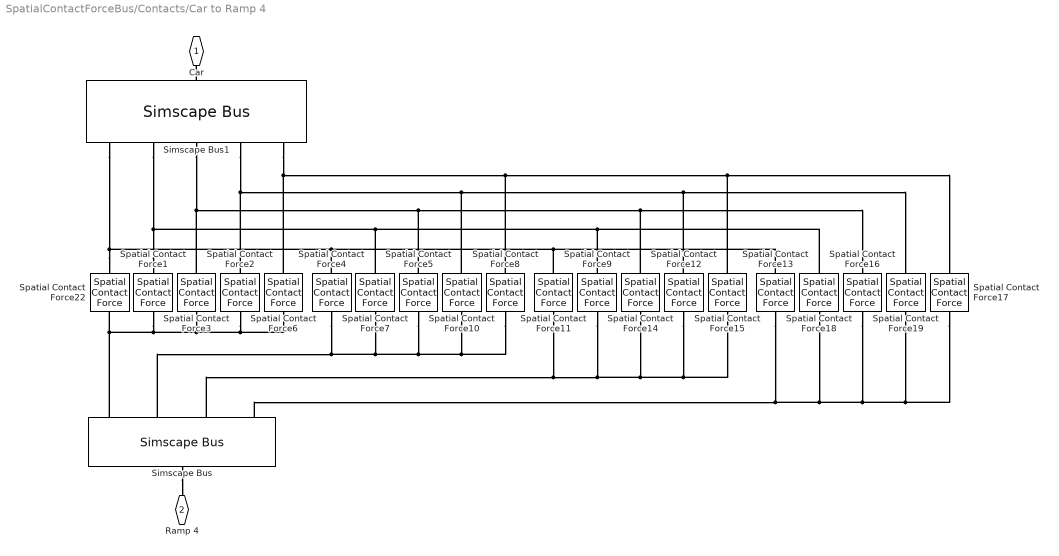
== system SpatialContactForceBus/Contacts/Car to Ramp 4 ==
  Simscape Bus : SimscapeBus  HierarchyStrings=Incline;BackStop;LeftRail;RightRail
  Simscape Bus1 : SimscapeBus  HierarchyStrings=Body;BackLeft;BackRight;FrontLeft;FrontRight
  Spatial Contact Force{1..19,22} (20 alike) : sm_lib/Forces and Torques/Spatial Contact Force  SenseSeparationDistance=off  NormalForceType=SmoothSpringDamper  NormalStiffness=k  NormalStiffnessUnits=N/m  NormalDamping=b  NormalDampingUnits=N/(m/s)  NormalTransitionRegionWidth=tau  NormalTransitionRegionWidthUnits=m  FrictionType=SmoothStickSlip  CoefficientOfStaticFriction=mus  CoefficientOfDynamicFriction=muk  FrictionalCriticalVelocity=cv  FrictionalCriticalVelocityUnits=m/s  SenseContactSignal=off  SensePenetrationDepth=off  SenseNormalVelocity=off  SenseTangentialVelocity=off  SensingForceTorqueDirection=BaseOnFollower  SensingForceTorqueResolutionFrame=ContactFrame  SenseNormalForce=off  SenseNormalForceMagnitude=off  SenseNormalTorque=off  SenseFrictionalForce=off  SenseFrictionalForceMagnitude=off  SenseFrictionalTorque=off  SenseTotalForce=off  SenseTotalTorque=off  SenseContactBaseRotation=off  SenseContactBaseTranslation=off  SenseContactFollowerRotation=off  SenseContactFollowerTranslation=off  ZeroCrossDetectContactStartAndEnd=off
  Car : PMIOPort  Side=Right
  Ramp 4 : PMIOPort  Port=2  Side=Left
  connections:
  Spatial Contact Force3/LConn1 -- Spatial Contact Force1/LConn1 -- Spatial Contact Force22/LConn1 -- Simscape Bus/LConn1 -- Spatial Contact Force6/LConn1 -- Spatial Contact Force2/LConn1
  Simscape Bus/LConn2 -- Spatial Contact Force4/LConn1 -- Spatial Contact Force7/LConn1 -- Spatial Contact Force5/LConn1 -- Spatial Contact Force8/LConn1 -- Spatial Contact Force10/LConn1
  Spatial Contact Force14/LConn1 -- Spatial Contact Force12/LConn1 -- Spatial Contact Force15/LConn1 -- Spatial Contact Force9/LConn1 -- Simscape Bus/LConn3 -- Spatial Contact Force11/LConn1
  Simscape Bus/LConn4 -- Spatial Contact Force13/LConn1 -- Spatial Contact Force16/LConn1 -- Spatial Contact Force19/LConn1 -- Spatial Contact Force17/LConn1 -- Spatial Contact Force18/LConn1
  Simscape Bus/RConn1 -- Ramp 4/RConn1
  Simscape Bus1/RConn1 -- Car/RConn1
  Spatial Contact Force22/RConn1 -- Simscape Bus1/LConn1 -- Spatial Contact Force4/RConn1 -- Spatial Contact Force13/RConn1 -- Spatial Contact Force11/RConn1
  Spatial Contact Force1/RConn1 -- Simscape Bus1/LConn2 -- Spatial Contact Force7/RConn1 -- Spatial Contact Force9/RConn1 -- Spatial Contact Force18/RConn1
  Simscape Bus1/LConn3 -- Spatial Contact Force16/RConn1 -- Spatial Contact Force14/RConn1 -- Spatial Contact Force5/RConn1 -- Spatial Contact Force3/RConn1
  Spatial Contact Force12/RConn1 -- Spatial Contact Force19/RConn1 -- Spatial Contact Force10/RConn1 -- Simscape Bus1/LConn4 -- Spatial Contact Force2/RConn1
  Spatial Contact Force15/RConn1 -- Spatial Contact Force17/RConn1 -- Spatial Contact Force8/RConn1 -- Spatial Contact Force6/RConn1 -- Simscape Bus1/LConn5
